simulink model "LedSwitchTask"  (R2018b)
settings: Solver=FixedStepDiscrete  StartTime=0.0  StopTime=inf  RelTol=1e-3
settings Model: Creator=dahroug  LastModifiedBy=dahroug
settings OptimizationCC: DefaultParameterBehavior=Inlined  EnhancedBackFolding=on  PassReuseOutputArgsAs=Individual arguments  OptimizeBlockOrder=speed  DifferentSizesBufferReuse=on  OptimizationCustomize=off
settings DebuggingCC: UnderspecifiedInitializationDetection=Classic  MergeDetectMultiDrivingBlocksExec=none  ParameterTunabilityLossMsg=error
settings ModelReferenceCC: PropagateSignalLabelsOutOfModel=off
settings SFSimCC: MATLABDynamicMemAlloc=off
settings RTWCC: SystemTargetFile=ert.tlc  GenCodeOnly=on  TemplateMakefile=ert_default_tmf  GenerateReport=on  IncludeHyperlinkInReport=on  LaunchReport=on  GenerateTraceInfo=on  GenerateTraceReport=on  GenerateTraceReportSl=on  GenerateTraceReportSf=on  GenerateTraceReportEml=on
settings CodeAppCC: ForceParamTrailComments=on  IgnoreCustomStorageClasses=off  OperatorAnnotations=on  SimulinkDataObjDesc=on  SFDataObjDesc=on  InsertBlockDesc=on
settings ERTTargetCC: TargetLangStandard=C99 (ISO)  GenerateSampleERTMain=on  InlinedParameterPlacement=NonHierarchical  ERTCustomFileTemplate=example_file_process.tlc

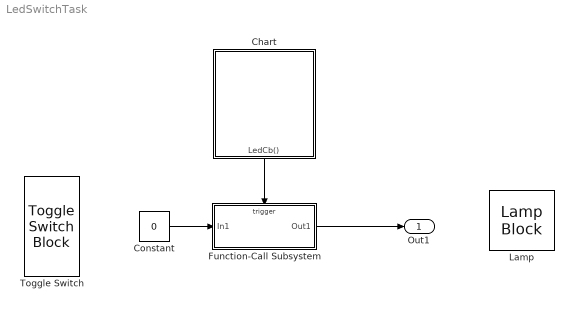
== system LedSwitchTask ==
  Chart : Stateflow chart  TreatAsAtomicUnit=on
  Constant : Constant  Value=0
  Function-Call Subsystem : Subsystem  TreatAsAtomicUnit=on
  Lamp : LampBlock  WebBlockId=9
  Toggle Switch : ToggleSwitchBlock  WebBlockId=8
      settings: Values={{'Off', 'On'}, [0 1]}
  Out1 : Outport
  wires:
  Constant/1 -> Function-Call Subsystem/1(In1)
  Function-Call Subsystem/1(Out1) -> Out1/1
  Chart/1(LedCb()) -> Function-Call Subsystem/Trigger

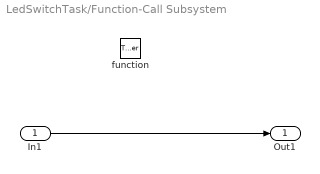
== system LedSwitchTask/Function-Call Subsystem ==
  In1 : Inport
  function : TriggerPort  TriggerType=function-call  VariantControl=Variant
  Out1 : Outport
  wires:
  In1/1 -> Out1/1

== stateflow chart LedSwitchTask/Chart ==
  state call
    en:
    du:
    ex:
  (default) -> call
  call -> call : [after (5,msec)]{LedCb;}
  events: LedCb output FUNCTION_CALL_EVENT
